simulink model "mech_flexible_string"  (Simulink 7.1)
settings: Solver=ode15s  StartTime=0.0  StopTime=1.4  FixedStep=0.005  RelTol=1e-2  AbsTol=1e-4
InitFcn:
  | %-----------------------------------------
  | % Defined in the block mask now. I have left it here because it can be
  | % used as a starting point of describing a material data file format
  | %-----------------------------------------
  | fBeamElement.material = 'Mild Steel';
  | 
  | % Beam element density (Kg/m^3)
  | fBeamElement.density = 7800;
  | 
  | % Beam element Youngs Modulus (N/m^2)
  | fBeamElement.youngsM = 210E6;
  | 
  | % Wire diameter
  | fBeamElement.diameter = 5E-4;
  | 
  | % Beam element length (m)
  | fBeamElement.length = 0.05;
  | 
  | % Length of CG vector along length of beam (m)
  | fBeamElement.cgLeng = fBeamElement.length/2;
  | 
  | % Beam element direction (along X direction it is [1 0 0])
  | fBeamElement.beamDir = [1 0 0];
  | 
  | % Beam element Mass Moment of Inertia (Kg/m^2)
  | fBeamElement.Inertia = [0.01 0 0;0 5.0 0;0 0 5.0]*0.5E-8;
  | 
  | % Damping coefficient
  | fBeamElement.matDamping = 0.5E-3;
  | %----------------------------------------
undefined symbols (not defined in the file or in its folder): sigbuilder_block
libraries: mech_flexible_element_lib x20, mblibv1 x7
Description:
  | Vibrating String
  | 
  | This model simulates a flexible string, plucked at the center with an initial force and then allowed to vibrate freely. The string is also subject to its own weight in gravity.
settings Model: Creator=arnav  LastModifiedBy=batserve  ExtModeAutoUpdateStatusClock=off
settings SolverCC: MaxOrder=2
settings DataIOCC: OutputOption=SpecifiedOutputTimes  OutputTimes=linspace(0,1.4,250)
settings DebuggingCC: SaveWithParameterizedLinksMsg=none  SignalResolutionControl=TryResolveAllWithWarning  SolverPrmCheckMsg=none  MultiTaskDSMMsg=warning  MultiTaskCondExecSysMsg=none  SigSpecEnsureSampleTimeMsg=none  StrictBusMsg=None
settings HardwareCC: TargetBitPerLong=64  TargetEndianess=LittleEndian  TargetWordSize=64  TargetHWDeviceType=MATLAB Host  ProdEqTarget=off
settings RTWCC: SystemTargetFile=rsim.tlc  TemplateMakefile=rsim_default_tmf  Description=Rapid Simulation Target  ProcessScript=rsim_make_rtw_hook  IncludeERTFirstTime=on
settings RSimTargetCC: TargetFcnLib=ansi_tfl_tmw.mat  TargetFunctionLibrary=ANSI_C  IsPILTarget=off  EnableShiftOperators=on  PortableWordSizes=off
settings SimMechanicsCC: WarnOnRedundantConstraints=off  VisOnUpdateDiagram=on  VisDuringSimulation=on  VisConfigFile=mech_flexible_string.mat

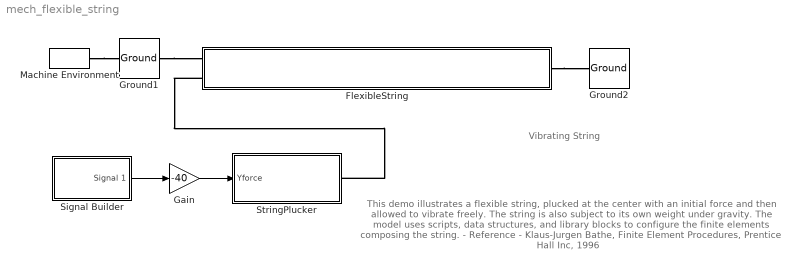
== system mech_flexible_string ==
  note: Vibrating String
  note: This demo illustrates a flexible string, plucked at the center
      | with an initial force and then allowed to vibrate freely.
      | The string is also subject to its own weight under gravity.
      |
      | The model uses scripts, data structures, and library blocks
      | to configure the finite elements composing the string.
      |
      | - Reference -
      |
      | Klaus-Jurgen Bathe, Finite Element Procedures, Prentice Hall Inc, 1996
  FlexibleString : Subsystem
  Gain : Gain  Gain=-40  ParameterDataType=sfix(16)  ParameterScaling=2^0  OutDataType=sfix(16)  OutScaling=2^0
  Ground1 : mblibv1/Bodies/Ground  DialogController=MECH.DynMechDlgSource  SystemSampleTime=-1  LeftPortType=env  RightPortType=workingframe  PhysicalDomain=Mechanical  DialogClass=GroundBlock  CoordPosition=[0 0 0]  CoordPositionUnits=m  StateVectorMgrId=-1  MachineId=[0 0]  ShowEnvPort=on
  Ground2 : mblibv1/Bodies/Ground  Orientation=left  DialogController=MECH.DynMechDlgSource  SystemSampleTime=-1  LeftPortType=env  RightPortType=workingframe  PhysicalDomain=Mechanical  DialogClass=GroundBlock  CoordPosition=[1 0 0]  CoordPositionUnits=m  StateVectorMgrId=-1  MachineId=[0 0]  ShowEnvPort=off
  Machine Environment : mblibv1/Bodies/Machine Environment  Tag=Factory ground  DialogController=MECH.DialogSource  SystemSampleTime=-1  PortType=env  PhysicalDomain=Mechanical  DialogTemplateClass=MECH.MachineEnvironment  SyncWhenCopied=off  Gravity=[0 -9.81 0]  GravityUnits=m/s^2  GravityAsSignal=off  Dimensionality=Auto-detect  AnalysisType=Forward dynamics  LinearAssemblyTolerance=1e-3  LinearAssemblyToleranceUnits=m  AngularAssemblyTolerance=1e-3  AngularAssemblyToleranceUnits=rad  ConstraintSolverType=Machine precision  ConstraintRelTolerance=1e-4  ConstraintAbsTolerance=1e-4  UseRobustSingularityHandling=off  RedundancyAnalysisToleranceType=Automatically select tolerance  RedundancyAnalysisTolerance=1e-14  StatePerturbationType=Fixed  PerturbationSize=1e-5  VisualizeMachine=on
  Signal Builder : Subsystem  Tag=STV Subsys  AncestorBlock=mech_flexible_element_lib/FlexibleElementActuator/Signal Builder  LoadFcn=sigbuilder_block('load');  StartFcn=sigbuilder_block('start');  StopFcn=sigbuilder_block('stop');  ClipboardFcn=sigbuilder_block('clipboard');  mask(Sigbuilder block){}
      mask help: Sigbuilder GUI
      mask init:
      | if ~strcmp(get_param(bdroot(gcbh),'SimulationStatus'),'stopped') tuvar = sigbuilder_block('maskInit'); end
      settings: CopyFcn=sigbuilder_block('copy');  DeleteFcn=sigbuilder_block('delete');  ModelCloseFcn=sigbuilder_block('modelClose');  PreSaveFcn=sigbuilder_block('preSave');  NameChangeFcn=sigbuilder_block('namechange');  OpenFcn=sigbuilder_block('open',[63.75 88.5 550.5 399.75 ]);  CloseFcn=sigbuilder_block('close');
      mask Display: plot(0,0,100,100,[10,10,40,40,10],[80,20,20,80,80],[40,10],[50,50], [40,27,10],[65,72,56],[40,25,25,10],[28,28,43,43]);
  StringPlucker : Subsystem
  wires:
  Signal Builder/1(Signal 1) -> Gain/1
  Gain/1 -> StringPlucker/1(Yforce)
  connections:
  Machine Environment/RConn1 -- Ground1/LConn1
  Ground1/RConn1 -- FlexibleString/LConn1
  FlexibleString/RConn1 -- Ground2/RConn1
  FlexibleString/LConn2 -- StringPlucker/RConn1

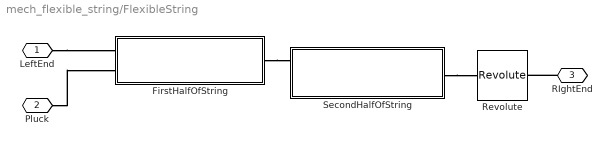
== system mech_flexible_string/FlexibleString ==
  FirstHalfOfString : Subsystem
  Revolute : mblibv1/Joints/Revolute  DialogController=MECH.DynMechDlgSource  PhysicalDomain=mechanical  SubClassName=Unknown  LeftPortType=blob  RightPortType=blob  LConnTagsString=__newl0  RConnTagsString=__newr0  NumSAPorts=0  CutJoint=off  MarkAsCut=off  Primitives=revolute  PrimitiveProps=R1$INERTIAL$[0 0 1]$revolute  DialogClass=JointBlock  R1Axis=[0 0 1]
  SecondHalfOfString : Subsystem
  LeftEnd : PMIOPort  Port=1  Side=Left
  Pluck : PMIOPort  Port=2  Side=Left
  RIghtEnd : PMIOPort  Orientation=left  Port=3  Side=Right
  connections:
  SecondHalfOfString/RConn1 -- Revolute/LConn1
  FirstHalfOfString/RConn1 -- SecondHalfOfString/LConn1
  LeftEnd/RConn1 -- FirstHalfOfString/LConn1
  Pluck/RConn1 -- FirstHalfOfString/LConn2
  RIghtEnd/RConn1 -- Revolute/RConn1

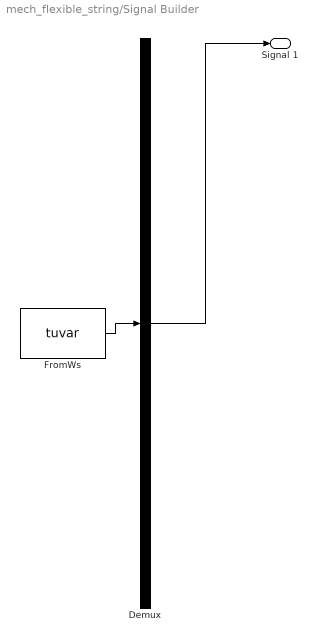
== system mech_flexible_string/Signal Builder ==
  Demux : Demux  Tag=STV Demux  Outputs=1
  FromWs : FromWorkspace  Tag=STV FromWs  VariableName=tuvar  SampleTime=0  SigBuilderData=DataTag2  VnvData=DataTag3
      SigBuilderData=|
      | channels.label = 'Signal 1'
      | channels.allXData = {[0 0.1 0.3 0.3 0.4 0.45 10]}
      | channels.allYData = {[0 0 1 1 1 0 0]}
      | common.afterFinalStr = 'Extrapolate'
      | common.sampleTime = 0
      | dataSet.timeRange = [0 10]
      | dataSet.name = 'Group 1'
  Signal 1 : Outport  Tag=STV Outport  OutDataType=sfix(16)  OutScaling=2^0
  wires:
  FromWs/1 -> Demux/1
  Demux/1 -> Signal 1/1

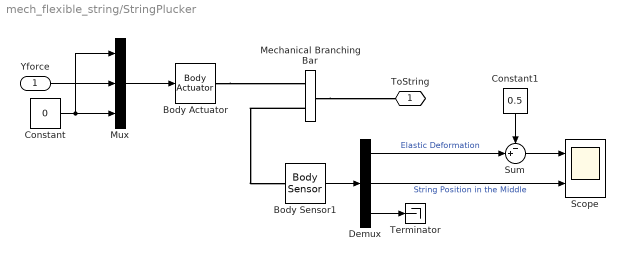
== system mech_flexible_string/StringPlucker ==
  Yforce : Inport  OutDataType=sfix(16)  OutScaling=2^0
  Body Actuator : mblibv1/Sensors &  Actuators/Body Actuator  DialogController=MECH.DynMechDlgSource  SystemSampleTime=-1  PhysicalDomain=Mechanical  PortType=blob  ActuationStyle=Force  AngleUnits=deg  ArcVelocityUnits=deg/s  ArcAccelerationUnits=deg/s^2  CoordPositionUnits=m  VelocityUnits=m/s  AccelerationUnits=m/s^2  ForceUnits=N  TorqueUnits=N-m  ActiveIO=on  Width=3  DialogClass=MechanicalActuatorBlock  ReferenceFrame=Absolute (World)  Angle=off  CoordPosition=on  Force=on  Torque=off
  Body Sensor1 : mblibv1/Sensors &  Actuators/Body Sensor  DialogController=MECH.DynMechDlgSource  SystemSampleTime=-1  PhysicalDomain=Mechanical  PortType=blob  Muxed=on  Pose=off  Angle=on  AngleUnits=deg  ArcVelocity=off  ArcVelocityUnits=rad/s  ArcAcceleration=off  ArcAccelerationUnits=deg/s^2  CoordPosition=on  CoordPositionUnits=m  Velocity=off  VelocityUnits=m/s  Acceleration=off  AccelerationUnits=m/s^2  Quaternion=on  QuaternionDT=off  QuaternionDDT=off  QuaternionUnits=off  OutputVector=[ 3 ]  ActiveIO=on  Width=3  DialogClass=MechanicalSensorBlock  ReferenceFrame=Absolute (World)
  Constant : Constant  Value=0  OutDataType=sfix(16)  OutScaling=2^0
  Constant1 : Constant  Orientation=down  Value=0.5  OutDataType=sfix(16)  OutScaling=2^0
  Demux : Demux  Outputs=3
  Mechanical Branching Bar : mblibv1/Utilities/Mechanical Branching Bar  Orientation=left  DialogController=MECH.DynMechDlgSource  PhysicalDomain=mechanical  SubClassName=Unknown  LeftPortType=blob  RightPortType=blob  LConnTagsString=_newl0  RConnTagsString=SA0|SA1  DialogClass=MechanicalBranchingBarBlock  NumSAPorts=2
  Mux : Mux  Inputs=3
  Scope : Scope  NumInputPorts=2
      settings: TimeRange=1.4  YMin=-0.02~-1  YMax=0.01~0.5
  Sum : Sum  Inputs=-+|  OutDataType=sfix(16)  OutScaling=2^0
  Terminator : Terminator
  ToString : PMIOPort  Orientation=left  Port=1  Side=Right
  wires:
  Constant/1 -> Mux/3, Mux/1
  Mux/1 -> Body Actuator/1
  Yforce/1 -> Mux/2
  Body Sensor1/1 -> Demux/1
  Demux/2 -> Scope/2  "String Position in the Middle"
  Demux/3 -> Terminator/1
  Demux/1 -> Sum/2  "Elastic Deformation"
  Sum/1 -> Scope/1
  Constant1/1 -> Sum/1
  connections:
  Body Actuator/RConn1 -- Mechanical Branching Bar/RConn1
  Mechanical Branching Bar/RConn2 -- Body Sensor1/LConn1
  Mechanical Branching Bar/LConn1 -- ToString/RConn1

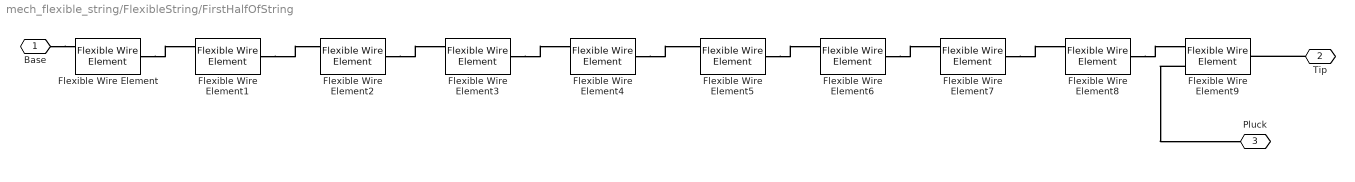
== system mech_flexible_string/FlexibleString/FirstHalfOfString ==
  Flexible Wire Element{,1..9} (10 alike) : mech_flexible_element_lib/Flexible Wire Element  SystemSampleTime=-1  material=Mild Steel  density=fBeamElement.density  wireDia=fBeamElement.diameter  length=fBeamElement.length  cgLeng=fBeamElement.cgLeng  beamDir=fBeamElement.beamDir  Inertia=fBeamElement.Inertia  youngsM=fBeamElement.youngsM  matDamping=fBeamElement.matDamping
  Base : PMIOPort  Port=1  Side=Left
  Tip : PMIOPort  Orientation=left  Port=2  Side=Right
  Pluck : PMIOPort  Orientation=left  Port=3  Side=Left
  connections:
  Flexible Wire Element/RConn1 -- Flexible Wire Element1/LConn1
  Flexible Wire Element1/RConn1 -- Flexible Wire Element2/LConn1
  Flexible Wire Element2/RConn1 -- Flexible Wire Element3/LConn1
  Flexible Wire Element3/RConn1 -- Flexible Wire Element4/LConn1
  Flexible Wire Element4/RConn1 -- Flexible Wire Element5/LConn1
  Flexible Wire Element5/RConn1 -- Flexible Wire Element6/LConn1
  Flexible Wire Element6/RConn1 -- Flexible Wire Element7/LConn1
  Flexible Wire Element7/RConn1 -- Flexible Wire Element8/LConn1
  Flexible Wire Element8/RConn1 -- Flexible Wire Element9/LConn1
  Base/RConn1 -- Flexible Wire Element/LConn1
  Tip/RConn1 -- Flexible Wire Element9/RConn1
  Flexible Wire Element9/LConn2 -- Pluck/RConn1

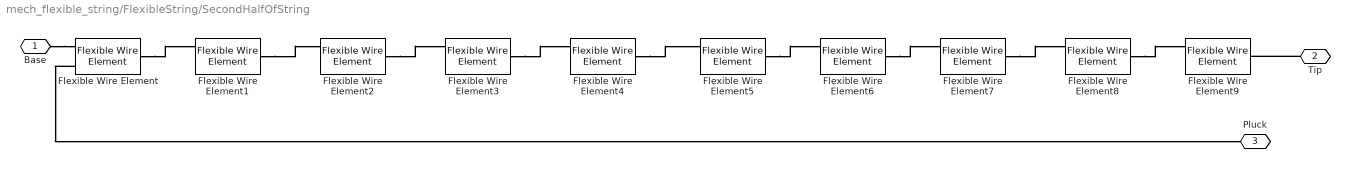
== system mech_flexible_string/FlexibleString/SecondHalfOfString ==
  Flexible Wire Element{,1..9} (10 alike) : mech_flexible_element_lib/Flexible Wire Element  SystemSampleTime=-1  material=Mild Steel  density=fBeamElement.density  wireDia=fBeamElement.diameter  length=fBeamElement.length  cgLeng=fBeamElement.cgLeng  beamDir=fBeamElement.beamDir  Inertia=fBeamElement.Inertia  youngsM=fBeamElement.youngsM  matDamping=fBeamElement.matDamping
  Base : PMIOPort  Port=1  Side=Left
  Tip : PMIOPort  Orientation=left  Port=2  Side=Right
  Pluck : PMIOPort  Orientation=left  Port=3  Side=Left
  connections:
  Tip/RConn1 -- Flexible Wire Element9/RConn1
  Base/RConn1 -- Flexible Wire Element/LConn1
  Flexible Wire Element8/RConn1 -- Flexible Wire Element9/LConn1
  Flexible Wire Element7/RConn1 -- Flexible Wire Element8/LConn1
  Flexible Wire Element6/RConn1 -- Flexible Wire Element7/LConn1
  Flexible Wire Element5/RConn1 -- Flexible Wire Element6/LConn1
  Flexible Wire Element4/RConn1 -- Flexible Wire Element5/LConn1
  Flexible Wire Element3/RConn1 -- Flexible Wire Element4/LConn1
  Flexible Wire Element2/RConn1 -- Flexible Wire Element3/LConn1
  Flexible Wire Element1/RConn1 -- Flexible Wire Element2/LConn1
  Flexible Wire Element/RConn1 -- Flexible Wire Element1/LConn1
  Flexible Wire Element/LConn2 -- Pluck/RConn1
